simulink model "Comparison_Simscape_SimHydraulics_Valve_Cylinder"  (R2014a)
settings: Solver=ode15s  StartTime=0.0  StopTime=10.0  RelTol=1e-6
InitFcn:
  | area_leak = 1e-9;
libraries: fl_lib x28, nesl_utility x8, sh_lib x2
Description:
  | Copyright 2014 The MathWorks, Inc.
settings Model: Creator=smiller  LastModifiedBy=smiller
settings DataIOCC: SignalLoggingSaveFormat=ModelDataLogs
settings OptimizationCC: ExpressionDepthLimit=2147483647  InitFltsAndDblsToZero=on
settings DebuggingCC: SaveWithParameterizedLinksMsg=none  UnderspecifiedInitializationDetection=Classic  FcnCallInpInsideContextMsg=UseLocalSettings  StateNameClashWarn=warning
settings GRTTargetCC: TargetFcnLib=ansi_tfl_tmw.mat  CombineOutputUpdateFcns=off  GRTInterface=on

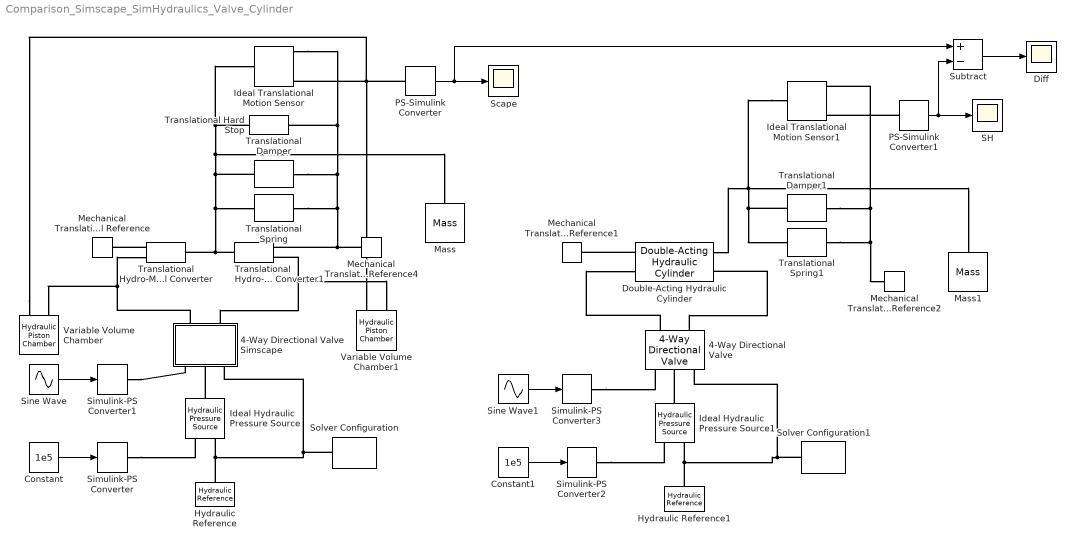
== system Comparison_Simscape_SimHydraulics_Valve_Cylinder ==
  4-Way Directional Valve : sh_lib/Valves/Directional Valves/4-Way Directional Valve  mdl_type=1  area_max=1e-05 m^2  opening_max=0.005 m  opening_tab="[  -0.002 0 0.005 0.015 ] m"  area_tab="[  1e-12 4e-12 1e-05 1.02e-05 ] m^2"  pressure_tab="[  -5e+06 -2e+06 2e+06 5e+06 ] Pa"  flow_rate_tab="[  -1e-12 -6e-14 6e+12 1e+11 ; -8e-08 -4e-08 4e+06 8e+06 ; -0.0025 -0.00103 0.001 0.0024 ; -0.00258 -0.001032 0.00106 0.00247 ; ] m^3/s"  interp_method=1  extrap_method=1  C_d=0.7  x_0_P_A=0 m  x_0_P_B=0 m  x_0_A_T=0 m  x_0_B_T=0 m  Re_cr=12  A_leak=area_leak m^2
  4-Way Directional Valve Simscape : Subsystem
  Constant : Constant  Value=1e5
  Constant1 : Constant  Value=1e5
  Diff : Scope
      settings: TimeRange=10  YMin=-3e-005  YMax=3e-005  SaveName=ScopeData2
  Double-Acting Hydraulic Cylinder : sh_lib/Hydraulic Cylinders/Double-Acting Hydraulic Cylinder  area_A=5e-04 m^2  area_B=5e-04 m^2  stroke=0.05 m  init_pos=0.025 m  dead_vol_A=1e-4 m^3  dead_vol_B=1e-4 m^3  init_pressure_A=0 Pa  init_pressure_B=0 Pa  k_sh=1.4  stiff=1e6 N/m  D=1500 N/(m/s)  or=1  or_sign=1
  Hydraulic Reference : fl_lib/Hydraulic/Hydraulic Elements/Hydraulic Reference
  Hydraulic Reference1 : fl_lib/Hydraulic/Hydraulic Elements/Hydraulic Reference
  Ideal Hydraulic Pressure Source : fl_lib/Hydraulic/Hydraulic Sources/Hydraulic Pressure Source
  Ideal Hydraulic Pressure Source1 : fl_lib/Hydraulic/Hydraulic Sources/Hydraulic Pressure Source
  Ideal Translational Motion Sensor : fl_lib/Mechanical/Mechanical Sensors/Ideal Translational Motion Sensor  offset=0 m
  Ideal Translational Motion Sensor1 : fl_lib/Mechanical/Mechanical Sensors/Ideal Translational Motion Sensor  offset=0 m
  Mass : fl_lib/Mechanical/Translational Elements/Mass  mass=1 kg  v_specify=on  v_priority=High  v=0 m/s  f_specify=off  f_priority=High  f=0 N
  Mass1 : fl_lib/Mechanical/Translational Elements/Mass  mass=1 kg  v_specify=on  v_priority=High  v=0 m/s  f_specify=off  f_priority=High  f=0 N
  Mechanical Translational Reference{,1..2,4} (4 alike) : fl_lib/Mechanical/Translational Elements/Mechanical Translational Reference
  PS-Simulink Converter : nesl_utility/PS-Simulink Converter  PhysicalDomain=network_engine_domain  SubClassName=ps_output  LeftPortType=input  RightPortType=output  PseudoPeriodic=off  Frequencies=[]  Unit=1  AffineConversion=off
  PS-Simulink Converter1 : nesl_utility/PS-Simulink Converter  PhysicalDomain=network_engine_domain  SubClassName=ps_output  LeftPortType=input  RightPortType=output  PseudoPeriodic=off  Frequencies=[]  Unit=1  AffineConversion=off
  SH : Scope
      settings: TimeRange=10  YMin=-0.03  YMax=0.03
  Scape : Scope
      settings: TimeRange=10  YMin=-0.03  YMax=0.03
  Simulink-PS Converter : nesl_utility/Simulink-PS Converter  PhysicalDomain=network_engine_domain  SubClassName=ps_input  LeftPortType=input  RightPortType=output  PseudoPeriodic=off  Frequencies=[]  NoiseDistribution=none  NoiseParameters=[]  Unit=1  AffineConversion=off  InputFiltering=off  SimscapeFilterOrder=1  InputFilterTimeConstant=.001  UdotUserProvided=0
  Simulink-PS Converter1 : nesl_utility/Simulink-PS Converter  PhysicalDomain=network_engine_domain  SubClassName=ps_input  LeftPortType=input  RightPortType=output  PseudoPeriodic=off  Frequencies=[]  NoiseDistribution=none  NoiseParameters=[]  Unit=m^2  AffineConversion=off  InputFiltering=off  SimscapeFilterOrder=1  InputFilterTimeConstant=.001  UdotUserProvided=0
  Simulink-PS Converter2 : nesl_utility/Simulink-PS Converter  PhysicalDomain=network_engine_domain  SubClassName=ps_input  LeftPortType=input  RightPortType=output  PseudoPeriodic=off  Frequencies=[]  NoiseDistribution=none  NoiseParameters=[]  Unit=1  AffineConversion=off  InputFiltering=off  SimscapeFilterOrder=1  InputFilterTimeConstant=.001  UdotUserProvided=0
  Simulink-PS Converter3 : nesl_utility/Simulink-PS Converter  PhysicalDomain=network_engine_domain  SubClassName=ps_input  LeftPortType=input  RightPortType=output  PseudoPeriodic=off  Frequencies=[]  NoiseDistribution=none  NoiseParameters=[]  Unit=m  AffineConversion=off  InputFiltering=off  SimscapeFilterOrder=1  InputFilterTimeConstant=.001  UdotUserProvided=0
  Sine Wave : Sin  Amplitude=1e-5  SampleTime=0
  Sine Wave1 : Sin  Amplitude=0.005  SampleTime=0
  Solver Configuration : nesl_utility/Solver Configuration  PhysicalDomain=network_engine_domain  SubClassName=solver  LeftPortType=input  RightPortType=generic  Accelerate=off  Tones=[]  Harmonics=[]  SimulateNoise=off  Profile=off  UseLocalSampling=off  EnableSwitchedLinearOptims=on  FrequencyDomain=off  UseCCode=off  RelTol=0.001  AbsTol=1e-06  MinStep=1e-09  ToWorkspace=off  DoDC=off  ResidualTolerance=1e-9  UseLocalSolver=off  LocalSolverChoice=NE_BACKWARD_EULER_ADVANCER  LocalSolverSampleTime=.001  DoFixedCost=off  MaxNonlinIter=12  MaxModeIter=2  LinearAlgebra=Sparse  DelaysMemoryBudget=1024  AutomaticFiltering=on  FilteringTimeConstant=0.001
  Solver Configuration1 : nesl_utility/Solver Configuration  PhysicalDomain=network_engine_domain  SubClassName=solver  LeftPortType=input  RightPortType=generic  Accelerate=off  Tones=[]  Harmonics=[]  SimulateNoise=off  Profile=off  UseLocalSampling=off  EnableSwitchedLinearOptims=on  FrequencyDomain=off  UseCCode=off  RelTol=0.001  AbsTol=1e-06  MinStep=1e-09  ToWorkspace=off  DoDC=off  ResidualTolerance=1e-9  UseLocalSolver=off  LocalSolverChoice=NE_BACKWARD_EULER_ADVANCER  LocalSolverSampleTime=.001  DoFixedCost=off  MaxNonlinIter=12  MaxModeIter=2  LinearAlgebra=Sparse  DelaysMemoryBudget=1024  AutomaticFiltering=on  FilteringTimeConstant=0.001
  Subtract : Sum  Inputs=+-
  Translational Hydro-Mechanical Converter : fl_lib/Hydraulic/Hydraulic Elements/Translational Hydro-Mechanical Converter  area=5e-04 m^2  or=1  compressibility=0  init_pos=0 m  V_dead=1e-4 m^3  k_sh=1.4  initial_pressure=0 Pa
  Translational Hydro-Mechanical Converter1 : fl_lib/Hydraulic/Hydraulic Elements/Translational Hydro-Mechanical Converter  area=5e-04 m^2  or=2  compressibility=0  init_pos=0 m  V_dead=1e-4 m^3  k_sh=1.4  initial_pressure=0 Pa
  Translational Damper : fl_lib/Mechanical/Translational Elements/Translational Damper  D=100 N/(m/s)  v_specify=off  v_priority=High  v=0 m/s  f_specify=off  f_priority=High  f=0 N
  Translational Damper1 : fl_lib/Mechanical/Translational Elements/Translational Damper  D=100 N/(m/s)  v_specify=off  v_priority=High  v=0 m/s  f_specify=off  f_priority=High  f=0 N
  Translational Hard Stop : fl_lib/Mechanical/Translational Elements/Translational Hard Stop  upper_bnd=0.025 m  lower_bnd=-0.025 m  stiff_up=1e+06 N/m  stiff_low=1e+06 N/m  D_up=1500 N/(m/s)  D_low=1500 N/(m/s)  v_specify=off  v_priority=High  v=0 m/s  f_specify=off  f_priority=High  f=0 N  x_specify=on  x_priority=High  x=0 m
  Translational Spring : fl_lib/Mechanical/Translational Elements/Translational Spring  spr_rate=1000 N/m  v_specify=off  v_priority=High  v=0 m/s  f_specify=off  f_priority=High  f=0 N  x_specify=on  x_priority=High  x=0 m
  Translational Spring1 : fl_lib/Mechanical/Translational Elements/Translational Spring  spr_rate=1000 N/m  v_specify=off  v_priority=High  v=0 m/s  f_specify=off  f_priority=High  f=0 N  x_specify=on  x_priority=High  x=0 m
  Variable Volume Chamber : fl_lib/Hydraulic/Hydraulic Elements/Hydraulic Piston Chamber  area=5e-04 m^2  init_pos=0 m  or=1  V_dead=1e-4 + 0.025*5e-4 m^3  k_sh=1.4  x_or=1  p_a=101325.0 Pa  chamber_flow_rate_specify=off  chamber_flow_rate_priority=High  chamber_flow_rate=1 m^3/s  pressure_specify=on  pressure_priority=High  pressure=0 Pa
  Variable Volume Chamber1 : fl_lib/Hydraulic/Hydraulic Elements/Hydraulic Piston Chamber  area=5e-04 m^2  init_pos=0 m  or=2  V_dead=1e-4 + 0.025*5e-4 m^3  k_sh=1.4  x_or=1  p_a=101325.0 Pa  chamber_flow_rate_specify=off  chamber_flow_rate_priority=High  chamber_flow_rate=1 m^3/s  pressure_specify=on  pressure_priority=High  pressure=0 Pa
  wires:
  Constant/1 -> Simulink-PS Converter/1
  Sine Wave/1 -> Simulink-PS Converter1/1
  PS-Simulink Converter/1 -> Scape/1, Subtract/1
  Sine Wave1/1 -> Simulink-PS Converter3/1
  Subtract/1 -> Diff/1
  Constant1/1 -> Simulink-PS Converter2/1
  PS-Simulink Converter1/1 -> SH/1, Subtract/2
  connections:
  Ideal Hydraulic Pressure Source/LConn1 -- 4-Way Directional Valve Simscape/LConn2
  Translational Hydro-Mechanical Converter/LConn1 -- Mechanical Translational Reference/LConn1
  Translational Hard Stop/RConn1 -- Ideal Translational Motion Sensor/RConn1 -- Translational Damper/RConn1 -- Translational Spring/RConn1 -- Mechanical Translational Reference4/LConn1 -- Translational Hydro-Mechanical Converter1/LConn1
  Simulink-PS Converter1/RConn1 -- 4-Way Directional Valve Simscape/LConn1
  Simulink-PS Converter/RConn1 -- Ideal Hydraulic Pressure Source/RConn1
  Variable Volume Chamber/LConn1 -- PS-Simulink Converter/LConn1 -- Ideal Translational Motion Sensor/RConn3 -- Variable Volume Chamber1/LConn1
  4-Way Directional Valve Simscape/RConn2 -- Translational Hydro-Mechanical Converter1/LConn2 -- Variable Volume Chamber1/LConn2
  4-Way Directional Valve Simscape/RConn1 -- Translational Hydro-Mechanical Converter/LConn2 -- Variable Volume Chamber/LConn2
  Hydraulic Reference/LConn1 -- Ideal Hydraulic Pressure Source/RConn2 -- 4-Way Directional Valve Simscape/LConn3 -- Solver Configuration/RConn1
  Translational Hard Stop/LConn1 -- Ideal Translational Motion Sensor/LConn1 -- Translational Damper/LConn1 -- Translational Spring/LConn1 -- Translational Hydro-Mechanical Converter1/RConn1 -- Translational Hydro-Mechanical Converter/RConn1 -- Mass/LConn1
  Ideal Translational Motion Sensor1/RConn1 -- Translational Spring1/RConn1 -- Mechanical Translational Reference2/LConn1 -- Translational Damper1/RConn1
  4-Way Directional Valve/RConn3 -- Solver Configuration1/RConn1 -- Ideal Hydraulic Pressure Source1/RConn2 -- Hydraulic Reference1/LConn1
  Ideal Translational Motion Sensor1/LConn1 -- Translational Damper1/LConn1 -- Translational Spring1/LConn1 -- Double-Acting Hydraulic Cylinder/RConn1 -- Mass1/LConn1
  4-Way Directional Valve/LConn2 -- Double-Acting Hydraulic Cylinder/RConn2
  4-Way Directional Valve/LConn1 -- Double-Acting Hydraulic Cylinder/LConn2
  Ideal Hydraulic Pressure Source1/LConn1 -- 4-Way Directional Valve/RConn2
  PS-Simulink Converter1/LConn1 -- Ideal Translational Motion Sensor1/RConn3
  Double-Acting Hydraulic Cylinder/LConn1 -- Mechanical Translational Reference1/LConn1
  Simulink-PS Converter2/RConn1 -- Ideal Hydraulic Pressure Source1/RConn1
  Simulink-PS Converter3/RConn1 -- 4-Way Directional Valve/RConn1

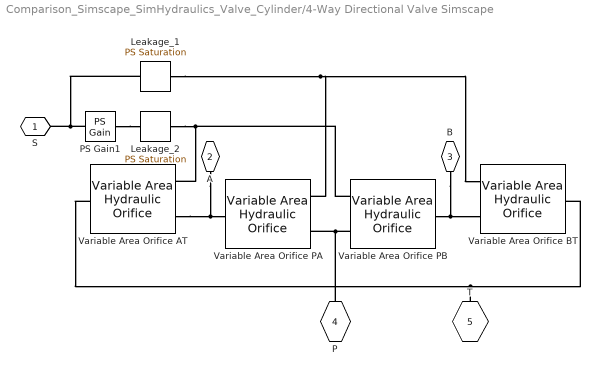
== system Comparison_Simscape_SimHydraulics_Valve_Cylinder/4-Way Directional Valve Simscape ==
  Leakage_1 : fl_lib/Physical Signals/Nonlinear Operators/PS Saturation  upper_limit=0.005 + area_leak  lower_limit=area_leak
  Leakage_2 : fl_lib/Physical Signals/Nonlinear Operators/PS Saturation  upper_limit=0.005 + area_leak  lower_limit=area_leak
  PS Gain1 : fl_lib/Physical Signals/Functions/PS Gain  gain=-1
  Variable Area Orifice AT : fl_lib/Hydraulic/Hydraulic Elements/Variable Area Hydraulic Orifice  C_d=0.7  Re_cr=12  min_area=1e-12 m^2  q_specify=off  q_priority=High  q=1 m^3/s  p_specify=off  p_priority=High  p=0 Pa
  Variable Area Orifice BT : fl_lib/Hydraulic/Hydraulic Elements/Variable Area Hydraulic Orifice  C_d=0.7  Re_cr=12  min_area=1e-12 m^2  q_specify=off  q_priority=High  q=1 m^3/s  p_specify=off  p_priority=High  p=0 Pa
  Variable Area Orifice PA : fl_lib/Hydraulic/Hydraulic Elements/Variable Area Hydraulic Orifice  C_d=0.7  Re_cr=12  min_area=1e-12 m^2  q_specify=off  q_priority=High  q=1 m^3/s  p_specify=off  p_priority=High  p=0 Pa
  Variable Area Orifice PB : fl_lib/Hydraulic/Hydraulic Elements/Variable Area Hydraulic Orifice  C_d=0.7  Re_cr=12  min_area=1e-12 m^2  q_specify=off  q_priority=High  q=1 m^3/s  p_specify=off  p_priority=High  p=0 Pa
  S : PMIOPort  Tag=PMCPort  Port=1  Side=Left
  A : PMIOPort  Tag=PMCPort  Port=2  Side=Right
  B : PMIOPort  Tag=PMCPort  Port=3  Side=Right
  P : PMIOPort  Tag=PMCPort  Port=4  Side=Left
  T : PMIOPort  Tag=PMCPort  Port=5  Side=Left
  connections:
  Variable Area Orifice PB/RConn1 -- Variable Area Orifice BT/LConn2 -- B/RConn1
  T/RConn1 -- Variable Area Orifice BT/RConn1 -- Variable Area Orifice AT/RConn1
  Variable Area Orifice PA/RConn1 -- Variable Area Orifice AT/LConn2 -- A/RConn1
  Variable Area Orifice PB/LConn2 -- Variable Area Orifice PA/LConn2 -- P/RConn1
  PS Gain1/LConn1 -- S/RConn1 -- Leakage_1/LConn1
  Leakage_1/RConn1 -- Variable Area Orifice PA/LConn1 -- Variable Area Orifice BT/LConn1
  Variable Area Orifice PB/LConn1 -- Leakage_2/RConn1 -- Variable Area Orifice AT/LConn1
  PS Gain1/RConn1 -- Leakage_2/LConn1
